simulink subsystem "example_ref_subsystem"  (R2023b)
settings: Solver=VariableStepAuto  StartTime=0.0  StopTime=10.0  RelTol=1e-3
settings Model: Creator=foregan  LastModifiedBy=foregan

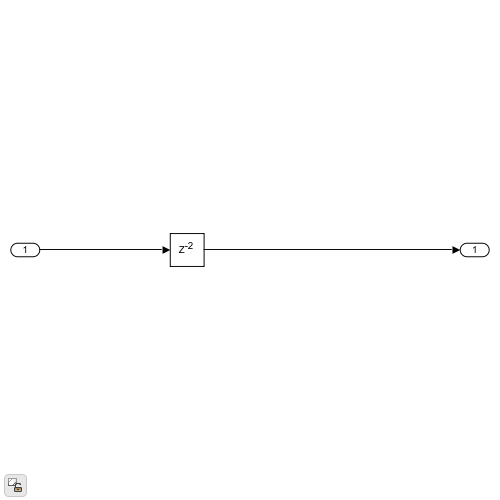
[thumbnail: Simulink's stored preview of the top-level diagram]
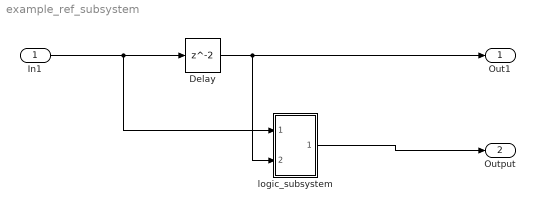
== system example_ref_subsystem ==
  In1 : Inport
  Delay : Delay
  logic_subsystem : Subsystem
  Out1 : Outport
  Output : Outport  Port=2
  wires:
  In1/1 -> Delay/1, logic_subsystem/1(In1)
  Delay/1 -> Out1/1, logic_subsystem/2(In2)
  logic_subsystem/1(Out1) -> Output/1

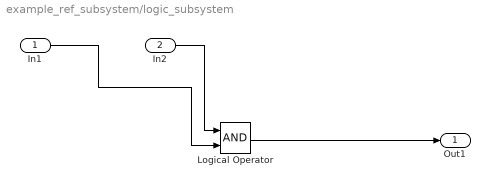
== system example_ref_subsystem/logic_subsystem ==
  In1 : Inport
  In2 : Inport  Port=2
  Logical Operator : Logic  AllPortsSameDT=off  OutDataTypeStr=boolean
  Out1 : Outport
  wires:
  Logical Operator/1 -> Out1/1
  In1/1 -> Logical Operator/2
  In2/1 -> Logical Operator/1
